simulink model "gimbal"  (R2019b)
settings: Solver=VariableStepAuto  StartTime=0.0  StopTime=10.0  RelTol=1e-3
InitFcn:
  | parameters
values from neighbouring files (symbols this model uses):
  ToDeg = 180/pi    (= 57.2957795131)    [parameters.m]    (also in test.m)
settings Model: Creator=Administrator  LastModifiedBy=Administrator

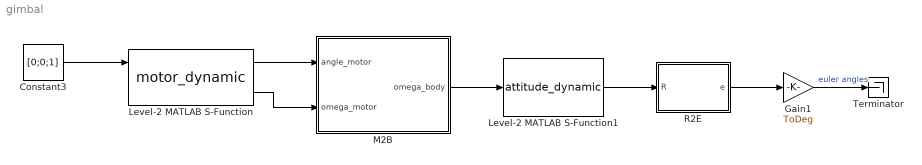
== system gimbal ==
  Constant3 : Constant  Value=[0;0;1]
  Gain1 : Gain  Gain=ToDeg
  Level-2 MATLAB S-Function : M-S-Function  FunctionName=motor_dynamic  Parameters=pa
  Level-2 MATLAB S-Function1 : M-S-Function  FunctionName=attitude_dynamic
  M2B : MATLAB Function  TreatAsAtomicUnit=on
  R2E : MATLAB Function  TreatAsAtomicUnit=on
  Terminator : Terminator
  wires:
  Level-2 MATLAB S-Function1/1 -> R2E/1(R)
  Gain1/1 -> Terminator/1  "euler angles"
  R2E/1(e) -> Gain1/1
  M2B/1(omega_body) -> Level-2 MATLAB S-Function1/1
  Level-2 MATLAB S-Function/1 -> M2B/1(angle_motor)
  Level-2 MATLAB S-Function/2 -> M2B/2(omega_motor)
  Constant3/1 -> Level-2 MATLAB S-Function/1

== matlab function gimbal/M2B ==
  data: angle_motor input; omega_motor input; omega_body output
function omega_body = fcn(angle_motor,omega_motor)

phi = angle_motor(1);
theta = angle_motor(2);
T = [cos(theta),0,-cos(phi)*sin(theta);
              0,1,            sin(phi);
     sin(theta),0, cos(phi)*cos(theta);];

omega_body = T*omega_motor;

== matlab function gimbal/R2E ==
  data: R input; e output
function e = fcn(R)

e = zeros(3,1);
e(1) = atan2(R(3,2),R(3,3));
e(2) = -asin(R(3,1));
e(3) = atan2(R(2,1),R(1,1));
